simulink model "task_extra"  (R2019b)
settings: Solver=VariableStepAuto  StartTime=0.0  StopTime=30  RelTol=1e-3
PostLoadFcn:
  | % Path for this models parameters
  | modelPath = which(bdroot);  % Simulink model's path
  | [modelDirPath, name, ext] = fileparts(modelPath); % Get the path to model's parent directory
  | paramsPath = modelDirPath+"\params4.mat"; % Path to model parameters
  | 
  | % Load model parameters from file if the file exists, otherwise, use default values
  | if isfile(paramsPath)
  |     params = load(paramsPath).params;
  | else
  |     params = [1000; 25; 0.1];
  | end
undefined symbols (not defined in the file): y_0
PostSaveFcn:
  | % Path for this models parameters
  | modelPath = which(bdroot);  % Simulink model's path
  | [modelDirPath, name, ext] = fileparts(modelPath); % Get the path to model's parent directory
  | paramsPath = modelDirPath+"\params4.mat"; % Path to model parameters
  | 
  | % Save params to file
  | save(paramsPath, 'params');
settings Model: EnablePacing=on  PacingRate=4  Creator=Muhammad Saud  LastModifiedBy=Muhammad Saud

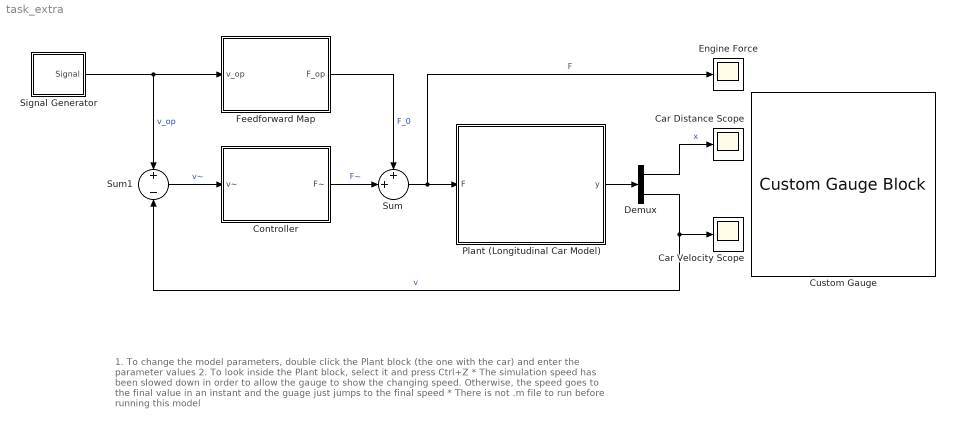
== system task_extra ==
  note: 1. To change the model parameters, double click the Plant block (the one with the car) and enter the parameter values
      | 2. To look inside the Plant block, select it and press Ctrl+Z
      |
      | * The simulation speed has been slowed down in order to allow the gauge to show the changing speed. Otherwise, the speed goes to the final value in an instant and the guage just jumps to the final speed
      | * There is not .m file to run before running this model
  Car Distance Scope : Scope
  Car Velocity Scope : Scope
  Controller : Subsystem
  Custom Gauge : CustomGaugeBlock  NeedleImage=data:image/svg+xml;base64,PD94bWwgdmVyc2lvbj0iMS4wIiBlbmNvZGluZz0idXRmLTgiPz4KPCEtLSBHZW5lcmF0b3I6IEFkb2JlIElsbHVzdHJhdG9yIDE5LjIuMSwgU1ZHIEV4cG9ydCBQbHVnLUluIC4gU1ZHIFZlcnNpb246IDYuMDAgQnVpbGQgMCkgIC0tPgo8c3ZnIHZlcnNpb249IjEuMSIgeG1sbnM9Imh0dHA6Ly93d3cudzMub3JnLzIwMDAvc3ZnIiB4bWxuczp4bGluaz0iaHR0cDovL3d3dy53My5vcmcvMTk5OS94bGluayIgeD0iMHB4IiB5PSIwcHgiCgkgdmlld0JveD0iMCAwIDIwMCA1MCIgc3R5bGU9ImVuYWJsZS1iYWNrZ3JvdW5kOm5ldyAw ...(+9940 chars)  NeedleXPos=0.3889630552760254  NeedleYPos=0.4825458547177911  NeedleHeight=0.10756162392620591  NeedleWidth=0.17719983286264462  NeedleInitialRotation=-59.94322499147643  BackgroundImage=data:image/svg+xml;base64,PD94bWwgdmVyc2lvbj0iMS4wIiBlbmNvZGluZz0iVVRGLTgiIHN0YW5kYWxvbmU9Im5vIj8+CjwhLS0gR2VuZXJhdG9yOiBBZG9iZSBJbGx1c3RyYXRvciAxOS4yLjEsIFNWRyBFeHBvcnQgUGx1Zy1JbiAuIFNWRyBWZXJzaW9uOiA2LjAwIEJ1aWxkIDApICAtLT4KCjxzdmcKICAgeG1sbnM6ZGM9Imh0dHA6Ly9wdXJsLm9yZy9kYy9lbGVtZW50cy8xLjEvIgogICB4bWxuczpjYz0iaHR0cDovL2NyZWF0aXZlY29tbW9ucy5vcmcvbnMjIgogICB4bWxuczpyZGY9Imh0dHA6Ly93d3cudzMub3JnLzE5OTkvMDIvMjItcmRmLXN5bnRh ...(+9660 chars)  GaugeMin=17  GaugeMax=27  GaugeArcDefined=true  GaugeArcRadius=0.1259502032464693  GaugeArcStrokeWidth=0.03683270138201725  GaugeArcRotation=240.5385250290321  GaugeArcRatio=0.8333333333333  GaugeArcTransparency=0  ValueArcColor=#1759b0  GaugeTickColor=#faf5c8  ScaleColorsJSON=[]  fixedAspectRatio=on  IsLinearGauge=false  GaugeTrackLeft=0.35  GaugeTrackTop=0.35  GaugeTrackHeight=0.1  GaugeTrackWidth=0.3  GaugeTrackRotation=0  ScaleMin=17
  Demux : Demux  Outputs=2
  Engine Force : Scope
  Feedforward Map : MATLAB Function  TreatAsAtomicUnit=on
  Plant (Longitudinal Car Model) : Subsystem  mask(Longitudinal Car Model){m=1000, b=25, cd=0.1, v_0=45, unit=Miles Per Hour}
      mask prompts: m "Enter the mass (kg) of the car"; b "Enter the ground friction coefficient (Nm/s)"; cd "Enter the drag coefficient (kg/m)"; v_0 "Enter the initial velocity of the car"; unit "Select units"
      mask help:
      | Defines and evaluates the longitudnal car dynamics:
      | F = m*a + b*v + cd*v^2
      mask init:
      | assignin('base', 'params', [m; b; cd]);
      mask Help: Please enter the parameter values corresponding to the mass (m) of the car, the coefficient of friction (b), and the drag coefficient (cd) in the block's dialog box.
      mask TypeOptions unit: Miles Per Hour | Meters Per Second
      mask DialogControl Container3 Prompt: Model Parameters
      mask DialogControl Container4 Prompt: Initial Velocity
      mask Display: image('$imagefile');
  Signal Generator : Subsystem
  Sum : Sum  Inputs=++|
  Sum1 : Sum  Inputs=+|-
  wires:
  Demux/2 -> Sum1/2, Car Velocity Scope/1  "v"
  Demux/1 -> Car Distance Scope/1  "x"
  Controller/1(F~) -> Sum/2  "F~"
  Sum/1 -> Engine Force/1, Plant (Longitudinal Car Model)/1(F)  "F"
  Plant (Longitudinal Car Model)/1(y) -> Demux/1
  Feedforward Map/1(F_op) -> Sum/1  "F_0"
  Sum1/1 -> Controller/1(v~)  "v~"
  Signal Generator/1(Signal) -> Sum1/1, Feedforward Map/1(v_op)  "v_op"

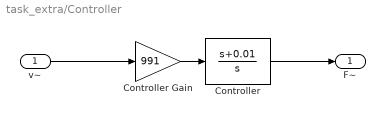
== system task_extra/Controller ==
  v~ : Inport
  Controller : TransferFcn  Numerator=[1 0.01]  Denominator=[1 0]
  Controller Gain : Gain  Gain=991
  F~ : Outport
  wires:
  Controller Gain/1 -> Controller/1
  v~/1 -> Controller Gain/1
  Controller/1 -> F~/1

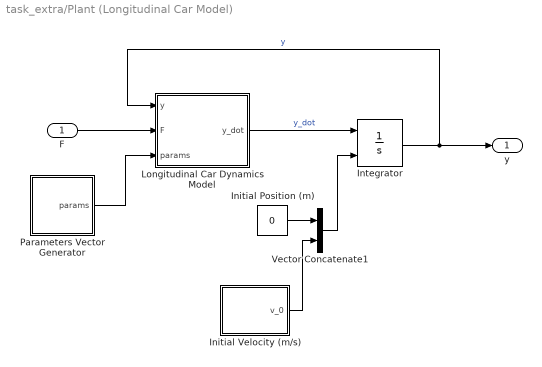
== system task_extra/Plant (Longitudinal Car Model) ==
  F : Inport
  Initial Position (m) : Constant  Value=0
  Initial Velocity (m/s) : Subsystem
  Integrator : Integrator  InitialConditionSource=external  InitialCondition=y_0
  Longitudinal Car Dynamics Model : MATLAB Function  TreatAsAtomicUnit=on
  Parameters Vector Generator : Subsystem
  Vector Concatenate1 : Concatenate
  y : Outport
  wires:
  Integrator/1 -> Longitudinal Car Dynamics Model/1(y), y/1  "y"
  F/1 -> Longitudinal Car Dynamics Model/2(F)
  Longitudinal Car Dynamics Model/1(y_dot) -> Integrator/1  "y_dot"
  Vector Concatenate1/1 -> Integrator/2
  Initial Position (m)/1 -> Vector Concatenate1/1
  Parameters Vector Generator/1(params) -> Longitudinal Car Dynamics Model/3(params)
  Initial Velocity (m/s)/1(v_0) -> Vector Concatenate1/2

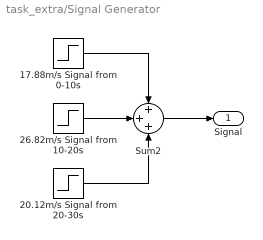
== system task_extra/Signal Generator ==
  17.88m/s Signal from 0-10s : Step  Time=0  After=17.88  SampleTime=0.01
  20.12m/s Signal from 20-30s : Step  Time=20  After=20.12-26.82  SampleTime=0.01
  26.82m/s Signal from 10-20s : Step  Time=10  After=26.82-17.88  SampleTime=0.01
  Sum2 : Sum  Inputs=+++
  Signal : Outport
  wires:
  26.82m/s Signal from 10-20s/1 -> Sum2/2
  20.12m/s Signal from 20-30s/1 -> Sum2/3
  17.88m/s Signal from 0-10s/1 -> Sum2/1
  Sum2/1 -> Signal/1

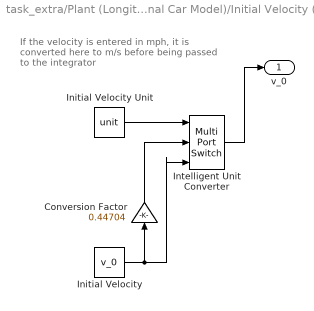
== system task_extra/Plant (Longitudinal Car Model)/Initial Velocity (m//s) ==
  note: If the velocity is entered in mph, it is converted here to m/s before being passed to the integrator
  Conversion Factor : Gain  Gain=0.44704
  Initial Velocity : Constant  Value=v_0
  Initial Velocity Unit : Constant  Value=unit
  Intelligent Unit Converter : MultiPortSwitch  Inputs=2
  v_0 : Outport
  wires:
  Initial Velocity Unit/1 -> Intelligent Unit Converter/1
  Initial Velocity/1 -> Intelligent Unit Converter/3, Conversion Factor/1
  Intelligent Unit Converter/1 -> v_0/1
  Conversion Factor/1 -> Intelligent Unit Converter/2

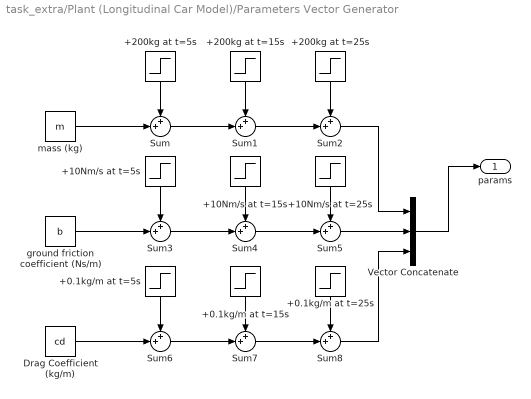
== system task_extra/Plant (Longitudinal Car Model)/Parameters Vector Generator ==
  +0.1kg/m at t=15s : Step  Time=15  After=0.1  SampleTime=0
  +0.1kg/m at t=25s : Step  Time=25  After=0.1  SampleTime=0
  +0.1kg/m at t=5s : Step  Time=5  After=0.1  SampleTime=0
  +10Nm/s at t=15s : Step  Time=15  After=10  SampleTime=0
  +10Nm/s at t=25s : Step  Time=25  After=10  SampleTime=0
  +10Nm/s at t=5s : Step  Time=5  After=10  SampleTime=0
  +200kg at t=15s : Step  Time=15  After=200  SampleTime=0
  +200kg at t=25s : Step  Time=25  After=200  SampleTime=0
  +200kg at t=5s : Step  Time=5  After=200  SampleTime=0
  Drag Coefficient (kg/m) : Constant  Value=cd
  Sum{,1..8} (9 alike) : Sum  Inputs=++|
  Vector Concatenate : Concatenate  NumInputs=3  Mode=Multidimensional array
  ground friction coefficient (Ns/m) : Constant  Value=b
  mass (kg) : Constant  Value=m
  params : Outport
  wires:
  Vector Concatenate/1 -> params/1
  Sum1/1 -> Sum2/2
  mass (kg)/1 -> Sum/2
  Sum/1 -> Sum1/2
  +200kg at t=5s/1 -> Sum/1
  +200kg at t=15s/1 -> Sum1/1
  +200kg at t=25s/1 -> Sum2/1
  Sum2/1 -> Vector Concatenate/1
  +10Nm/s at t=25s/1 -> Sum5/1
  Sum4/1 -> Sum5/2
  Sum3/1 -> Sum4/2
  +10Nm/s at t=15s/1 -> Sum4/1
  +10Nm/s at t=5s/1 -> Sum3/1
  ground friction coefficient (Ns/m)/1 -> Sum3/2
  Sum5/1 -> Vector Concatenate/2
  +0.1kg/m at t=15s/1 -> Sum7/1
  Sum7/1 -> Sum8/2
  Sum6/1 -> Sum7/2
  +0.1kg/m at t=25s/1 -> Sum8/1
  +0.1kg/m at t=5s/1 -> Sum6/1
  Drag Coefficient (kg/m)/1 -> Sum6/2
  Sum8/1 -> Vector Concatenate/3

== matlab function task_extra/Feedforward Map ==
  data: v_op input; F_op output; params parameter
function F_op = feedforward_map(v_op, params)
    %% Specifies mapping from nominal velocity to nominal force
    % Inputs:
    % -------
    % v_op: The nominal velocity (velocity at equilibrium point)
    % params: A vector of system parameters
    %         It is a 3-dimensional column vector of the form:
    %         [mass; ground_friction-coefficient; drag_coefficient]
    %
    % Output:
    % -------
    % F_op: The nominal force (force at equilibrium point)
    
    % Unpacking Parameters
    m = params(1)
    b = params(2)
    cd = params(3)
    
    % Defining feedforward mapping from v_op to F_op
    F_op = b*v_op + cd*v_op^2;

end % end feedforward_map function

== matlab function task_extra/Plant (Longitudinal Car Model)/Longitudinal Car Dynamics Model ==
  data: y input; y_dot output; F input; params input
function y_dot = car(y, F, params)
    %% This subroutine defines the longitudal car dynamics
    % Inputs
    % ------
    % y: State vector
    %    It is a 2-dimensional column vector of the form:
    %    [distance; car_velocity]
    % F: Input force (acting on the car)
    % params: A vector of model parameters
    %         It is a 3-dimensional column vector of the form:
    %         [mass; ground_friction-coefficient; drag_coefficient]
    %
    % Outputs
    % -------
    % y_dot: Time derivative of the state vector
    %        It has the same dimension as the state vector (y) and is of
    %        the form:
    %        [car_velocity; acceleration];
    
    % Unpacking parameters
    m = params(1);
    b = params(2);
    cd = params(3);
    
    % Defining the ODEs describing system's dynamics
    y_dot_1 = y(2); % ODE defining car velocity
    y_dot_2 = (F-b*y(2)-cd*y(2)^2)/m; % ODE defining car acceleration
    
    % Pack the differentiated states into a vector
    y_dot = [y_dot_1; y_dot_2];
    
end % end car subroutine
